simulink model "test2"  (R2018a)
settings: Solver=VariableStepAuto  StartTime=0.0  StopTime=50  RelTol=1e-3
undefined symbols (not defined in the file): x20
settings Model: Creator=john  LastModifiedBy=john
settings SolverCC: AlgebraicLoopSolver=LineSearch

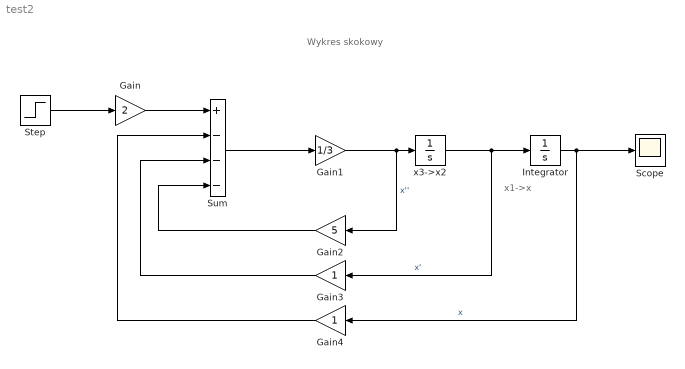
== system test2 ==
  note: Wykres skokowy
  note: x1->x
  Gain : Gain  Gain=2
  Gain1 : Gain  Gain=1/3
  Gain2 : Gain  Gain=5
  Gain3 : Gain
  Gain4 : Gain
  Integrator : Integrator
  Scope : Scope
  Step : Step  SampleTime=0
  Sum : Sum  Inputs=+---
  "x3->x2 " : Integrator  InitialCondition=x20
  wires:
  Gain/1 -> Sum/1
  Sum/1 -> Gain1/1
  Gain1/1 -> Gain2/1, "x3->x2 "/1  "x''"
  "x3->x2 "/1 -> Gain3/1, Integrator/1  "x'"
  Integrator/1 -> Gain4/1, Scope/1  "x"
  Gain2/1 -> Sum/4
  Gain3/1 -> Sum/3
  Gain4/1 -> Sum/2
  Step/1 -> Gain/1
